simulink model "wlan_agc"  (Simulink 7.8)
settings: Solver=VariableStepDiscrete  SolverMode=SingleTasking  StartTime=0.0  StopTime=1e4  RelTol=1e-3
PostLoadFcn:
  | wlan_agc_init
InitFcn:
  | wlan_agc_init
StartFcn:
  | wlan_agc_init
undefined symbols (not defined in the file): gcbh, PHY_CONFIG_PKT_DET_CORR_THRESH, PHY_CONFIG_PKT_DET_ENERGY_THRESH, PHY_CONFIG_PKT_DET_MIN_DURR, xlBlockLoadCallback, xlGetNormalizedPeriod
libraries: xbsIndex_r4 x991, xbsEDKLib_r4 x1, simulink x1
(part 5 of 7)

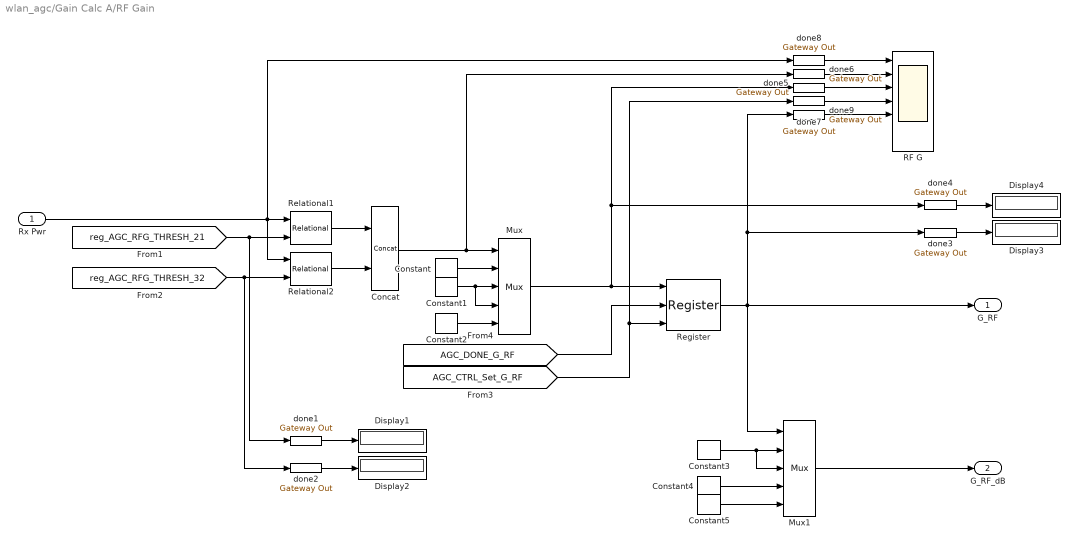
== system wlan_agc/Gain Calc A/RF Gain ==
  Rx Pwr : Inport
  Concat : xbsIndex_r4/Concat  num_inputs=2  dbl_ovrd=off  block_type=concat
  Constant : xbsIndex_r4/Constant  const=3  gui_display_data_type=Fixed-point  arith_type=Unsigned  n_bits=2  bin_pt=0  preci_type=Single  exp_width=8  frac_width=24  explicit_period=off  period=1  equ=P=C  opselect=C  inp2=PCIN>>17  opr=+  inp1=P  carry=CIN  dbl_ovrd=off  block_type=constant
  Constant1 : xbsIndex_r4/Constant  const=2  gui_display_data_type=Fixed-point  arith_type=Unsigned  n_bits=2  bin_pt=0  preci_type=Single  exp_width=8  frac_width=24  explicit_period=off  period=1  equ=P=C  opselect=C  inp2=PCIN>>17  opr=+  inp1=P  carry=CIN  dbl_ovrd=off  block_type=constant
  Constant2 : xbsIndex_r4/Constant  const=1  gui_display_data_type=Fixed-point  arith_type=Unsigned  n_bits=2  bin_pt=0  preci_type=Single  exp_width=8  frac_width=24  explicit_period=off  period=1  equ=P=C  opselect=C  inp2=PCIN>>17  opr=+  inp1=P  carry=CIN  dbl_ovrd=off  block_type=constant
  Constant3 : xbsIndex_r4/Constant  const=0  gui_display_data_type=Fixed-point  arith_type=Unsigned  n_bits=6  bin_pt=0  preci_type=Single  exp_width=8  frac_width=24  explicit_period=off  period=1  equ=P=C  opselect=C  inp2=PCIN>>17  opr=+  inp1=P  carry=CIN  dbl_ovrd=off  block_type=constant
  Constant4 : xbsIndex_r4/Constant  const=15  gui_display_data_type=Fixed-point  arith_type=Unsigned  n_bits=6  bin_pt=0  preci_type=Single  exp_width=8  frac_width=24  explicit_period=off  period=1  equ=P=C  opselect=C  inp2=PCIN>>17  opr=+  inp1=P  carry=CIN  dbl_ovrd=off  block_type=constant
  Constant5 : xbsIndex_r4/Constant  const=34  gui_display_data_type=Fixed-point  arith_type=Unsigned  n_bits=6  bin_pt=0  preci_type=Single  exp_width=8  frac_width=24  explicit_period=off  period=1  equ=P=C  opselect=C  inp2=PCIN>>17  opr=+  inp1=P  carry=CIN  dbl_ovrd=off  block_type=constant
  Display{1..4} (4 alike) : Display
  Mux : xbsIndex_r4/Mux  inputs=4  en=off  latency=0  precision=Full  arith_type=Unsigned  n_bits=16  bin_pt=14  quantization=Truncate  overflow=Wrap  dbl_ovrd=off  block_type=mux
  Mux1 : xbsIndex_r4/Mux  inputs=4  en=off  latency=0  precision=Full  arith_type=Unsigned  n_bits=16  bin_pt=14  quantization=Truncate  overflow=Wrap  dbl_ovrd=off  block_type=mux
  RF G : Scope  NumInputPorts=7
      settings: TimeRange=10000  YMin=-1~-1~0~0~0~-40~-1  YMax=1~1~0.8~0.2~80~0~1  SaveName=ScopeData5
  Register : xbsIndex_r4/Register  init=3  rst=on  en=on  dbl_ovrd=off  block_type=register
  Relational1 : xbsIndex_r4/Relational  mode=a>=b  en=off  latency=0  dbl_ovrd=off  block_type=relational
  Relational2 : xbsIndex_r4/Relational  mode=a>=b  en=off  latency=0  dbl_ovrd=off  block_type=relational
  done{1..9} (9 alike) : xbsIndex_r4/Gateway Out  inherit_from_input=off  hdl_port=off  timing_constraint=None  locs_specified=off  LOCs={}  UseAsDAC=off  DACChannel='1'  block_type=gatewayout
      settings: infoedit="Gateway out block.  Converts Xilinx fixed point inputs into ouputs of type Simulink integer, double, or fixed point.<P><P>Hardware notes:  In hardware these blocks become top level output ports or are discarded, depending on how they are configured."  xl_area=[0 0 0 0 1 0 0]  block_version=VER_STRING_GOES_HERE
  G_RF : Outport
  G_RF_dB : Outport  Port=2
  wires:
  Rx Pwr/1 -> Relational1/1, Relational2/1, done8/1
  [reg_AGC_RFG_THRESH_21] -> Relational1/2, done1/1
  Relational1/1 -> Concat/1
  [reg_AGC_RFG_THRESH_32] -> Relational2/2, done2/1
  Relational2/1 -> Concat/2
  Concat/1 -> Mux/1, done6/1
  Constant/1 -> Mux/2
  Constant1/1 -> Mux/3, Mux/4
  Constant2/1 -> Mux/5
  Mux/1 -> Register/1, done4/1, done5/1
  [AGC_DONE_G_RF] -> Register/2
  Register/1 -> G_RF/1, Mux1/1, done3/1, done9/1
  [AGC_CTRL_Set_G_RF] -> Register/3, done7/1
  Constant3/1 -> Mux1/2, Mux1/3
  Constant4/1 -> Mux1/4
  Constant5/1 -> Mux1/5
  Mux1/1 -> G_RF_dB/1
  done1/1 -> Display1/1
  done2/1 -> Display2/1
  done3/1 -> Display3/1
  done4/1 -> Display4/1
  done8/1 -> RF G/1
  done6/1 -> RF G/2
  done5/1 -> RF G/3
  done7/1 -> RF G/4
  done9/1 -> RF G/5

== system wlan_agc/Gain Calc A/RSSI Avg ==
  note: Flush recursive sum whenever sum
      | length changes. Otherwise let it run
      | (overflow is impossible, and lower
      | latency here is helpful to AGC timing)
  RSSI : Inport
  ASR : xbsIndex_r4/Addressable Shift Register  infer_latency=on  depth=2  initVector=[0]  en=off  dbl_ovrd=off  use_behavioral_HDL=off  Optimization=Resource  use_rpm=off  block_type=addrsr
      settings: infoedit="Delay of configurable length.  Any element in the delay line can be addressed and driven onto the output port.<br><br>Hardware notes: This block is implemented using SRL16s. If Virtex-4 or Spartan-3 device is used, multiple SRLC16s are cascaded together."  block_version=VER_STRING_GOES_HERE
  Accumulator : xbsIndex_r4/Accumulator  operation=Add  n_bits=16  overflow=Flag as error  scale=1  rst=on  infoeditControl=reset for floating point data type must be asserted for a minimum of 2 cycles  hasbypass=off  en=off  latency=0  dbl_ovrd=off  msb_inp=100  msb=100  lsb=-100  use_behavioral_HDL=on  implementation=Fabric  block_type=accum
      settings: block_version=VER_STRING_GOES_HERE
  AddSub : xbsIndex_r4/AddSub  mode=Subtraction  use_carryin=off  use_carryout=off  en=off  latency=0  precision=Full  arith_type=Unsigned  n_bits=10  bin_pt=0  quantization=Truncate  overflow=Wrap  dbl_ovrd=off  use_behavioral_HDL=off  hw_selection=Fabric  pipelined=off  use_rpm=on  block_type=addsub
      settings: block_version=VER_STRING_GOES_HERE
  Constant : xbsIndex_r4/Constant  const=0  gui_display_data_type=Fixed-point  arith_type=Unsigned  n_bits=2  bin_pt=0  preci_type=Single  exp_width=8  frac_width=24  explicit_period=off  period=1  equ=P=C  opselect=C  inp2=PCIN>>17  opr=+  inp1=P  carry=CIN  dbl_ovrd=off  block_type=constant
  Constant1 : xbsIndex_r4/Constant  const=1  gui_display_data_type=Fixed-point  arith_type=Unsigned  n_bits=2  bin_pt=0  preci_type=Single  exp_width=8  frac_width=24  explicit_period=off  period=1  equ=P=C  opselect=C  inp2=PCIN>>17  opr=+  inp1=P  carry=CIN  dbl_ovrd=off  block_type=constant
  Constant2 : xbsIndex_r4/Constant  const=3  gui_display_data_type=Fixed-point  arith_type=Unsigned  n_bits=3  bin_pt=0  preci_type=Single  exp_width=8  frac_width=24  explicit_period=off  period=1  equ=P=C  opselect=C  inp2=PCIN>>17  opr=+  inp1=P  carry=CIN  dbl_ovrd=off  block_type=constant
  Constant3 : xbsIndex_r4/Constant  const=7  gui_display_data_type=Fixed-point  arith_type=Unsigned  n_bits=3  bin_pt=0  preci_type=Single  exp_width=8  frac_width=24  explicit_period=off  period=1  equ=P=C  opselect=C  inp2=PCIN>>17  opr=+  inp1=P  carry=CIN  dbl_ovrd=off  block_type=constant
  Convert1 : xbsIndex_r4/Convert  gui_display_data_type=Fixed-point  arith_type=Unsigned  n_bits=10  bin_pt=0  float_type=Single  exp_bits=8  fraction_bits=24  quantization=Truncate  overflow=Saturate  en=off  latency=0  dbl_ovrd=off  pipeline=off  block_type=convert
      settings: block_version=10.1.3
  Down Sample1 : xbsIndex_r4/Down Sample  sample_ratio=16  sample_phase="Last Value of Frame  (most efficient)"  en=off  latency=1  dbl_ovrd=off  block_type=dsamp
  Mux : xbsIndex_r4/Mux  inputs=4  en=off  latency=0  precision=Full  arith_type=Unsigned  n_bits=16  bin_pt=14  quantization=Truncate  overflow=Wrap  dbl_ovrd=off  block_type=mux
  Mux1 : xbsIndex_r4/Mux  inputs=4  en=off  latency=0  precision=Full  arith_type=Unsigned  n_bits=16  bin_pt=14  quantization=Truncate  overflow=Wrap  dbl_ovrd=off  block_type=mux
  RSSI Avg : Scope  NumInputPorts=7
      settings: TimeRange=10000  YMin=0~0~0~0~0~-1~-1  YMax=1000~2~1~4000~1000~1~1  SaveName=ScopeData2
  Register : xbsIndex_r4/Register  init=0  rst=on  en=off  dbl_ovrd=off  block_type=register
      settings: block_version=VER_STRING_GOES_HERE
  Reset : Subsystem
  Shift : xbsIndex_r4/Shift  shift_dir=Right  shift_bits=1  en=off  latency=0  precision=Full  arith_type="Signed  (2's comp)"  n_bits=16  bin_pt=14  quantization=Truncate  overflow=Wrap  dbl_ovrd=off  block_type=shift
  Shift1 : xbsIndex_r4/Shift  shift_dir=Right  shift_bits=2  en=off  latency=0  precision=Full  arith_type="Signed  (2's comp)"  n_bits=16  bin_pt=14  quantization=Truncate  overflow=Wrap  dbl_ovrd=off  block_type=shift
  Shift2 : xbsIndex_r4/Shift  shift_dir=Right  shift_bits=3  en=off  latency=0  precision=Full  arith_type="Signed  (2's comp)"  n_bits=16  bin_pt=14  quantization=Truncate  overflow=Wrap  dbl_ovrd=off  block_type=shift
  done{2..6} (5 alike) : xbsIndex_r4/Gateway Out  inherit_from_input=off  hdl_port=off  timing_constraint=None  locs_specified=off  LOCs={}  UseAsDAC=off  DACChannel='1'  block_type=gatewayout
      settings: infoedit="Gateway out block.  Converts Xilinx fixed point inputs into ouputs of type Simulink integer, double, or fixed point.<P><P>Hardware notes:  In hardware these blocks become top level output ports or are discarded, depending on how they are configured."  xl_area=[0 0 0 0 1 0 0]  block_version=VER_STRING_GOES_HERE
  avg : Outport
  wires:
  ASR/1 -> AddSub/2
  AddSub/1 -> Accumulator/1
  Register/1 -> ASR/1, AddSub/1
  RSSI/1 -> Register/1, done4/1
  Accumulator/1 -> Mux1/2, Shift/1, Shift1/1, Shift2/1, done3/1
  Constant/1 -> Mux/2
  Constant1/1 -> Mux/3
  Constant2/1 -> Mux/4
  [reg_RSSI_AVG_LEN_SEL] -> Down Sample1/1, Mux1/1
  Constant3/1 -> Mux/5
  Mux/1 -> ASR/2
  Shift/1 -> Mux1/3
  Shift1/1 -> Mux1/4
  Shift2/1 -> Mux1/5
  Mux1/1 -> Convert1/1
  Convert1/1 -> avg/1, done6/1
  Down Sample1/1 -> Mux/1, Reset/1(Start), done2/1
  Reset/1(Rst) -> Accumulator/2, Register/2, done5/1
  done4/1 -> RSSI Avg/1
  done2/1 -> RSSI Avg/2
  done6/1 -> RSSI Avg/5
  done5/1 -> RSSI Avg/3
  done3/1 -> RSSI Avg/4
  ? -> RSSI Avg/6
  ? -> RSSI Avg/7

== system wlan_agc/Gain Calc B/BB gain ==
  G_RF_dB : Inport
  P_IN_RSSI : Inport  Port=2
  IQ_dBv : Inport  Port=3
  AddSub : xbsIndex_r4/AddSub  mode=Subtraction  use_carryin=off  use_carryout=off  en=off  latency=1  precision=User Defined  arith_type="Signed  (2's comp)"  n_bits=8  bin_pt=0  quantization=Truncate  overflow=Wrap  dbl_ovrd=off  use_behavioral_HDL=off  hw_selection=Fabric  pipelined=off  block_type=addsub
  AddSub1 : xbsIndex_r4/AddSub  mode=Subtraction  use_carryin=off  use_carryout=off  en=off  latency=1  precision=User Defined  arith_type="Signed  (2's comp)"  n_bits=8  bin_pt=0  quantization=Truncate  overflow=Wrap  dbl_ovrd=off  use_behavioral_HDL=off  hw_selection=Fabric  pipelined=off  block_type=addsub
  AddSub2 : xbsIndex_r4/AddSub  mode=Subtraction  use_carryin=off  use_carryout=off  en=off  latency=0  precision=User Defined  arith_type="Signed  (2's comp)"  n_bits=8  bin_pt=0  quantization=Truncate  overflow=Wrap  dbl_ovrd=off  use_behavioral_HDL=off  hw_selection=Fabric  pipelined=off  block_type=addsub
  AddSub3 : xbsIndex_r4/AddSub  mode=Addition  use_carryin=off  use_carryout=off  en=off  latency=1  precision=User Defined  arith_type="Signed  (2's comp)"  n_bits=8  bin_pt=0  quantization=Truncate  overflow=Wrap  dbl_ovrd=off  use_behavioral_HDL=off  hw_selection=Fabric  pipelined=off  block_type=addsub
  AddSub4 : xbsIndex_r4/AddSub  mode=Subtraction  use_carryin=off  use_carryout=off  en=off  latency=0  precision=User Defined  arith_type="Signed  (2's comp)"  n_bits=8  bin_pt=0  quantization=Truncate  overflow=Wrap  dbl_ovrd=off  use_behavioral_HDL=off  hw_selection=Fabric  pipelined=off  block_type=addsub
  Convert1 : xbsIndex_r4/Convert  gui_display_data_type=Fixed-point  arith_type=Unsigned  n_bits=5  bin_pt=0  float_type=Single  exp_bits=8  fraction_bits=24  quantization=Truncate  overflow=Saturate  en=off  latency=0  dbl_ovrd=off  pipeline=off  block_type=convert
  Convert2 : xbsIndex_r4/Convert  gui_display_data_type=Fixed-point  arith_type=Unsigned  n_bits=5  bin_pt=0  float_type=Single  exp_bits=8  fraction_bits=24  quantization=Truncate  overflow=Saturate  en=off  latency=0  dbl_ovrd=off  pipeline=off  block_type=convert
  Mux : xbsIndex_r4/Mux  inputs=3  en=off  latency=0  precision=Full  arith_type=Unsigned  n_bits=16  bin_pt=14  quantization=Truncate  overflow=Wrap  dbl_ovrd=off  block_type=mux
  Shift : xbsIndex_r4/Shift  shift_dir=Right  shift_bits=1  en=off  latency=0  precision=Full  arith_type="Signed  (2's comp)"  n_bits=16  bin_pt=14  quantization=Truncate  overflow=Wrap  dbl_ovrd=off  block_type=shift
  Shift1 : xbsIndex_r4/Shift  shift_dir=Right  shift_bits=1  en=off  latency=0  precision=Full  arith_type="Signed  (2's comp)"  n_bits=16  bin_pt=14  quantization=Truncate  overflow=Wrap  dbl_ovrd=off  block_type=shift
  G_BB : Outport
  wires:
  [reg_AGC_V_DB_ADJ] -> AddSub4/2
  IQ_dBv/1 -> AddSub4/1
  [AGC_CTRL_G_BB_SEL] -> Mux/1
  AddSub4/1 -> AddSub2/2
  P_IN_RSSI/1 -> AddSub/2
  Mux/1 -> G_BB/1
  G_RF_dB/1 -> AddSub1/2
  Convert2/1 -> Mux/4
  Convert1/1 -> Mux/3
  Shift1/1 -> Convert2/1
  AddSub3/1 -> Shift1/1
  AddSub2/1 -> AddSub3/1
  Shift/1 -> Convert1/1
  AddSub1/1 -> AddSub3/2, Shift/1
  AddSub/1 -> AddSub1/1
  [reg_AGC_TARGET_PWR] -> AddSub2/1, AddSub/1
  [reg_AGC_INIT_G_BB] -> Mux/2

== system wlan_agc/Gain Calc B/Capture & Convert ==
  note: Shift slope-adjusted value by gain-dependent
      | offset (top-center plot on pg 16 of MAX2829 ds)
  G_RF : Inport
  RSSI : Inport  Port=2
  AddSub : xbsIndex_r4/AddSub  mode=Subtraction  use_carryin=off  use_carryout=off  en=off  latency=1  precision=User Defined  arith_type="Signed  (2's comp)"  n_bits=8  bin_pt=0  quantization=Truncate  overflow=Flag as error  dbl_ovrd=off  use_behavioral_HDL=off  hw_selection=Fabric  pipelined=off  block_type=addsub
  Constant : xbsIndex_r4/Constant  const=1/15  gui_display_data_type=Fixed-point  arith_type=Unsigned  n_bits=12  bin_pt=12  preci_type=Single  exp_width=8  frac_width=24  explicit_period=off  period=1  equ=P=C  opselect=C  inp2=PCIN>>17  opr=+  inp1=P  carry=CIN  dbl_ovrd=off  block_type=constant
  Constant1 : xbsIndex_r4/Constant  const=100  gui_display_data_type=Fixed-point  arith_type=Unsigned  n_bits=7  bin_pt=0  preci_type=Single  exp_width=8  frac_width=24  explicit_period=off  period=1  equ=P=C  opselect=C  inp2=PCIN>>17  opr=+  inp1=P  carry=CIN  dbl_ovrd=off  block_type=constant
  Constant2 : xbsIndex_r4/Constant  const=85  gui_display_data_type=Fixed-point  arith_type=Unsigned  n_bits=7  bin_pt=0  preci_type=Single  exp_width=8  frac_width=24  explicit_period=off  period=1  equ=P=C  opselect=C  inp2=PCIN>>17  opr=+  inp1=P  carry=CIN  dbl_ovrd=off  block_type=constant
  Constant3 : xbsIndex_r4/Constant  const=70  gui_display_data_type=Fixed-point  arith_type=Unsigned  n_bits=7  bin_pt=0  preci_type=Single  exp_width=8  frac_width=24  explicit_period=off  period=1  equ=P=C  opselect=C  inp2=PCIN>>17  opr=+  inp1=P  carry=CIN  dbl_ovrd=off  block_type=constant
  Display : Display
  Display1 : Display
  Display2 : Display
  Mult : xbsIndex_r4/Mult  precision=User Defined  arith_type=Unsigned  n_bits=11  bin_pt=4  quantization=Truncate  overflow=Wrap  en=off  latency=1  dbl_ovrd=off  use_behavioral_HDL=off  opt=Speed  use_embedded=on  optimum_pipeline=off  pipeline=on  use_rpm=on  placement_style=Triangular  block_type=mult
  Mux1 : xbsIndex_r4/Mux  inputs=4  en=off  latency=0  precision=Full  arith_type=Unsigned  n_bits=16  bin_pt=14  quantization=Truncate  overflow=Wrap  dbl_ovrd=off  block_type=mux
  RSSI Calc : Scope  NumInputPorts=7
      settings: TimeRange=10000  YMin=-1~-1~0~0~0~-40~-1  YMax=1~1~0.8~0.2~80~0~1  SaveName=ScopeData7
  Register : xbsIndex_r4/Register  init=3  rst=on  en=on  dbl_ovrd=off  block_type=register
  done{1..8} (8 alike) : xbsIndex_r4/Gateway Out  inherit_from_input=off  hdl_port=off  timing_constraint=None  locs_specified=off  LOCs={}  UseAsDAC=off  DACChannel='1'  block_type=gatewayout
      settings: infoedit="Gateway out block.  Converts Xilinx fixed point inputs into ouputs of type Simulink integer, double, or fixed point.<P><P>Hardware notes:  In hardware these blocks become top level output ports or are discarded, depending on how they are configured."  xl_area=[0 0 0 0 1 0 0]  block_version=VER_STRING_GOES_HERE
  Rx Pwr (dBm) : Outport
  wires:
  done8/1 -> RSSI Calc/5
  done6/1 -> RSSI Calc/4
  done3/1 -> RSSI Calc/3
  done5/1 -> RSSI Calc/2
  done7/1 -> RSSI Calc/1
  done2/1 -> Display2/1
  done1/1 -> Display1/1
  done4/1 -> Display/1
  G_RF/1 -> Mux1/1
  [reg_AGC_RSSI_CALIB_G3] -> Mux1/5
  [reg_AGC_RSSI_CALIB_G2] -> Mux1/4
  [reg_AGC_RSSI_CALIB_G1] -> Mux1/3, Mux1/2
  AddSub/1 -> done8/1, done2/1, Rx Pwr (dBm)/1
  Mux1/1 -> done6/1, AddSub/2
  Mult/1 -> done4/1, AddSub/1
  Constant/1 -> Mult/2
  Register/1 -> done3/1, done1/1, Mult/1
  RSSI/1 -> done7/1, Register/1
  [AGC_RESET] -> Register/2
  [AGC_CTRL_Capture_RSSI] -> done5/1, Register/3

== system wlan_agc/Gain Calc B/IQ Mag ==
  I : Inport
  Q : Inport  Port=2
  Valid : Inport  Port=3
  AddSub : xbsIndex_r4/AddSub  mode=Addition  use_carryin=off  use_carryout=off  en=off  latency=0  precision=User Defined  arith_type=Unsigned  n_bits=20  bin_pt=19  quantization=Truncate  overflow=Flag as error  dbl_ovrd=off  use_behavioral_HDL=off  hw_selection=Fabric  pipelined=off  block_type=addsub
  Delay : xbsIndex_r4/Delay  rst=off  infoeditControl=Selection of Reset will increase slice count due to use of real FFs and instead of SRLs  en=off  latency=1  dbl_ovrd=off  reg_retiming=off  block_type=delay
  Mult : xbsIndex_r4/Mult  precision=User Defined  arith_type=Unsigned  n_bits=20  bin_pt=20  quantization=Truncate  overflow=Saturate  en=off  latency=1  dbl_ovrd=off  use_behavioral_HDL=off  opt=Speed  use_embedded=on  optimum_pipeline=off  pipeline=on  use_rpm=on  placement_style=Triangular  block_type=mult
  Mult1 : xbsIndex_r4/Mult  precision=User Defined  arith_type=Unsigned  n_bits=20  bin_pt=20  quantization=Truncate  overflow=Saturate  en=off  latency=1  dbl_ovrd=off  use_behavioral_HDL=off  opt=Speed  use_embedded=on  optimum_pipeline=off  pipeline=on  use_rpm=on  placement_style=Triangular  block_type=mult
  ROM : xbsIndex_r4/ROM  depth=2^11  initVector=5*log10(linspace(2^-11, 2, 2048))  distributed_mem=Block RAM  rst=off  init_reg=0  en=off  latency=1  gui_display_data_type=Fixed-point  arith_type="Signed  (2's comp)"  n_bits=14  bin_pt=8  preci_type=Single  exp_width=8  frac_width=24  dbl_ovrd=off  optimize=Area  use_rpm=on  block_type=sprom
  Register : xbsIndex_r4/Register  init=0  rst=on  en=on  dbl_ovrd=off  block_type=register
  Reinterpret : xbsIndex_r4/Reinterpret  force_arith_type=off  arith_type=Unsigned  force_bin_pt=on  bin_pt=0  block_type=reinterpret
  Running Sum : Subsystem
  V_DB : Scope  NumInputPorts=7
      settings: TimeRange=10000  YMin=-0.75~-0.75~0~0~0~-17.5~-1  YMax=0.75~0.75~0.35~0.125~125~0~1  SaveName=ScopeData4
  done{1..7} (7 alike) : xbsIndex_r4/Gateway Out  inherit_from_input=off  hdl_port=off  timing_constraint=None  locs_specified=off  LOCs={}  UseAsDAC=off  DACChannel='1'  block_type=gatewayout
      settings: infoedit="Gateway out block.  Converts Xilinx fixed point inputs into ouputs of type Simulink integer, double, or fixed point.<P><P>Hardware notes:  In hardware these blocks become top level output ports or are discarded, depending on how they are configured."  xl_area=[0 0 0 0 1 0 0]  block_version=VER_STRING_GOES_HERE
  IQ_dBv : Outport
  wires:
  done7/1 -> V_DB/7
  done6/1 -> V_DB/6
  done5/1 -> V_DB/5
  done3/1 -> V_DB/4
  done1/1 -> V_DB/3
  done2/1 -> V_DB/2
  done4/1 -> V_DB/1
  Reinterpret/1 -> done5/1, ROM/1
  Register/1 -> IQ_dBv/1
  [AGC_DONE_G_BB] -> Register/2
  [AGC_CTRL_Capture_V_DB] -> done7/1, Register/3
  ROM/1 -> done6/1, Register/1
  AddSub/1 -> done1/1, Running Sum/2(D)
  Mult1/1 -> AddSub/2
  Mult/1 -> AddSub/1
  Q/1 -> done2/1, Mult1/1, Mult1/2
  Running Sum/1(Sum) -> done3/1, Reinterpret/1
  Valid/1 -> Delay/1
  I/1 -> done4/1, Mult/2, Mult/1
  Delay/1 -> Running Sum/1(En)

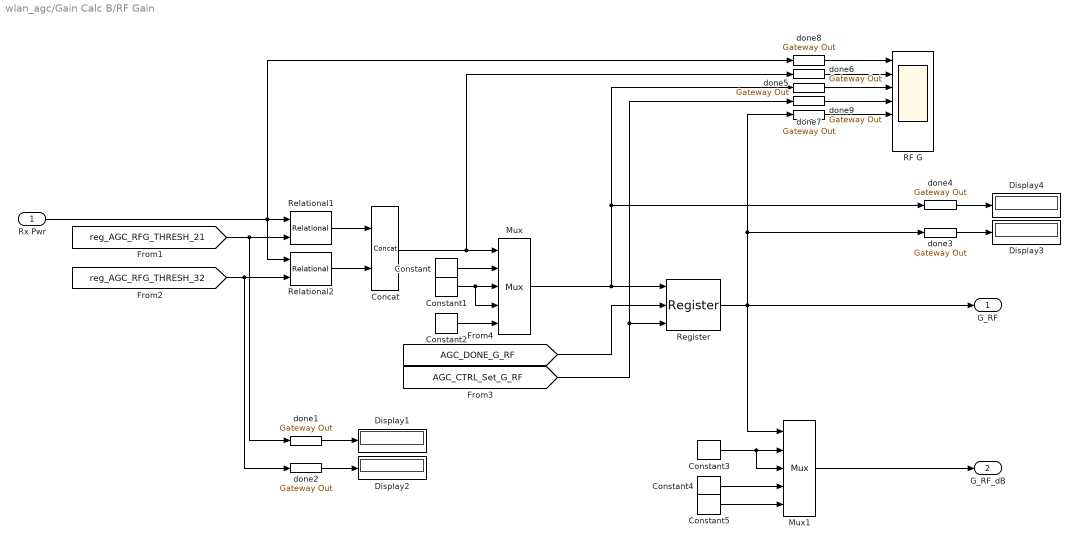
== system wlan_agc/Gain Calc B/RF Gain ==
  Rx Pwr : Inport
  Concat : xbsIndex_r4/Concat  num_inputs=2  dbl_ovrd=off  block_type=concat
  Constant : xbsIndex_r4/Constant  const=3  gui_display_data_type=Fixed-point  arith_type=Unsigned  n_bits=2  bin_pt=0  preci_type=Single  exp_width=8  frac_width=24  explicit_period=off  period=1  equ=P=C  opselect=C  inp2=PCIN>>17  opr=+  inp1=P  carry=CIN  dbl_ovrd=off  block_type=constant
  Constant1 : xbsIndex_r4/Constant  const=2  gui_display_data_type=Fixed-point  arith_type=Unsigned  n_bits=2  bin_pt=0  preci_type=Single  exp_width=8  frac_width=24  explicit_period=off  period=1  equ=P=C  opselect=C  inp2=PCIN>>17  opr=+  inp1=P  carry=CIN  dbl_ovrd=off  block_type=constant
  Constant2 : xbsIndex_r4/Constant  const=1  gui_display_data_type=Fixed-point  arith_type=Unsigned  n_bits=2  bin_pt=0  preci_type=Single  exp_width=8  frac_width=24  explicit_period=off  period=1  equ=P=C  opselect=C  inp2=PCIN>>17  opr=+  inp1=P  carry=CIN  dbl_ovrd=off  block_type=constant
  Constant3 : xbsIndex_r4/Constant  const=0  gui_display_data_type=Fixed-point  arith_type=Unsigned  n_bits=6  bin_pt=0  preci_type=Single  exp_width=8  frac_width=24  explicit_period=off  period=1  equ=P=C  opselect=C  inp2=PCIN>>17  opr=+  inp1=P  carry=CIN  dbl_ovrd=off  block_type=constant
  Constant4 : xbsIndex_r4/Constant  const=15  gui_display_data_type=Fixed-point  arith_type=Unsigned  n_bits=6  bin_pt=0  preci_type=Single  exp_width=8  frac_width=24  explicit_period=off  period=1  equ=P=C  opselect=C  inp2=PCIN>>17  opr=+  inp1=P  carry=CIN  dbl_ovrd=off  block_type=constant
  Constant5 : xbsIndex_r4/Constant  const=34  gui_display_data_type=Fixed-point  arith_type=Unsigned  n_bits=6  bin_pt=0  preci_type=Single  exp_width=8  frac_width=24  explicit_period=off  period=1  equ=P=C  opselect=C  inp2=PCIN>>17  opr=+  inp1=P  carry=CIN  dbl_ovrd=off  block_type=constant
  Display{1..4} (4 alike) : Display
  Mux : xbsIndex_r4/Mux  inputs=4  en=off  latency=0  precision=Full  arith_type=Unsigned  n_bits=16  bin_pt=14  quantization=Truncate  overflow=Wrap  dbl_ovrd=off  block_type=mux
  Mux1 : xbsIndex_r4/Mux  inputs=4  en=off  latency=0  precision=Full  arith_type=Unsigned  n_bits=16  bin_pt=14  quantization=Truncate  overflow=Wrap  dbl_ovrd=off  block_type=mux
  RF G : Scope  NumInputPorts=7
      settings: TimeRange=10000  YMin=-1~-1~0~0~0~-40~-1  YMax=1~1~0.8~0.2~80~0~1  SaveName=ScopeData5
  Register : xbsIndex_r4/Register  init=3  rst=on  en=on  dbl_ovrd=off  block_type=register
  Relational1 : xbsIndex_r4/Relational  mode=a>=b  en=off  latency=0  dbl_ovrd=off  block_type=relational
  Relational2 : xbsIndex_r4/Relational  mode=a>=b  en=off  latency=0  dbl_ovrd=off  block_type=relational
  done{1..9} (9 alike) : xbsIndex_r4/Gateway Out  inherit_from_input=off  hdl_port=off  timing_constraint=None  locs_specified=off  LOCs={}  UseAsDAC=off  DACChannel='1'  block_type=gatewayout
      settings: infoedit="Gateway out block.  Converts Xilinx fixed point inputs into ouputs of type Simulink integer, double, or fixed point.<P><P>Hardware notes:  In hardware these blocks become top level output ports or are discarded, depending on how they are configured."  xl_area=[0 0 0 0 1 0 0]  block_version=VER_STRING_GOES_HERE
  G_RF : Outport
  G_RF_dB : Outport  Port=2
  wires:
  done9/1 -> RF G/5
  done7/1 -> RF G/4
  done5/1 -> RF G/3
  done6/1 -> RF G/2
  done8/1 -> RF G/1
  done4/1 -> Display4/1
  done3/1 -> Display3/1
  done2/1 -> Display2/1
  done1/1 -> Display1/1
  Mux1/1 -> G_RF_dB/1
  Constant5/1 -> Mux1/5
  Constant4/1 -> Mux1/4
  Constant3/1 -> Mux1/3, Mux1/2
  [AGC_CTRL_Set_G_RF] -> done7/1, Register/3
  Register/1 -> done9/1, done3/1, Mux1/1, G_RF/1
  [AGC_DONE_G_RF] -> Register/2
  Mux/1 -> done5/1, done4/1, Register/1
  Constant2/1 -> Mux/5
  Constant1/1 -> Mux/4, Mux/3
  Constant/1 -> Mux/2
  Concat/1 -> done6/1, Mux/1
  Relational2/1 -> Concat/2
  [reg_AGC_RFG_THRESH_32] -> done2/1, Relational2/2
  Relational1/1 -> Concat/1
  [reg_AGC_RFG_THRESH_21] -> done1/1, Relational1/2
  Rx Pwr/1 -> done8/1, Relational2/1, Relational1/1

== system wlan_agc/Gain Calc B/RSSI Avg ==
  note: Flush recursive sum whenever sum
      | length changes. Otherwise let it run
      | (overflow is impossible, and lower
      | latency here is helpful to AGC timing)
  RSSI : Inport
  ASR : xbsIndex_r4/Addressable Shift Register  infer_latency=on  depth=2  initVector=[0]  en=off  dbl_ovrd=off  use_behavioral_HDL=off  Optimization=Resource  use_rpm=off  block_type=addrsr
      settings: infoedit="Delay of configurable length.  Any element in the delay line can be addressed and driven onto the output port.<br><br>Hardware notes: This block is implemented using SRL16s. If Virtex-4 or Spartan-3 device is used, multiple SRLC16s are cascaded together."  block_version=VER_STRING_GOES_HERE
  Accumulator : xbsIndex_r4/Accumulator  operation=Add  n_bits=16  overflow=Flag as error  scale=1  rst=on  infoeditControl=reset for floating point data type must be asserted for a minimum of 2 cycles  hasbypass=off  en=off  latency=0  dbl_ovrd=off  msb_inp=100  msb=100  lsb=-100  use_behavioral_HDL=on  implementation=Fabric  block_type=accum
      settings: block_version=VER_STRING_GOES_HERE
  AddSub : xbsIndex_r4/AddSub  mode=Subtraction  use_carryin=off  use_carryout=off  en=off  latency=0  precision=Full  arith_type=Unsigned  n_bits=10  bin_pt=0  quantization=Truncate  overflow=Wrap  dbl_ovrd=off  use_behavioral_HDL=off  hw_selection=Fabric  pipelined=off  use_rpm=on  block_type=addsub
      settings: block_version=VER_STRING_GOES_HERE
  Constant : xbsIndex_r4/Constant  const=0  gui_display_data_type=Fixed-point  arith_type=Unsigned  n_bits=2  bin_pt=0  preci_type=Single  exp_width=8  frac_width=24  explicit_period=off  period=1  equ=P=C  opselect=C  inp2=PCIN>>17  opr=+  inp1=P  carry=CIN  dbl_ovrd=off  block_type=constant
  Constant1 : xbsIndex_r4/Constant  const=1  gui_display_data_type=Fixed-point  arith_type=Unsigned  n_bits=2  bin_pt=0  preci_type=Single  exp_width=8  frac_width=24  explicit_period=off  period=1  equ=P=C  opselect=C  inp2=PCIN>>17  opr=+  inp1=P  carry=CIN  dbl_ovrd=off  block_type=constant
  Constant2 : xbsIndex_r4/Constant  const=3  gui_display_data_type=Fixed-point  arith_type=Unsigned  n_bits=3  bin_pt=0  preci_type=Single  exp_width=8  frac_width=24  explicit_period=off  period=1  equ=P=C  opselect=C  inp2=PCIN>>17  opr=+  inp1=P  carry=CIN  dbl_ovrd=off  block_type=constant
  Constant3 : xbsIndex_r4/Constant  const=7  gui_display_data_type=Fixed-point  arith_type=Unsigned  n_bits=3  bin_pt=0  preci_type=Single  exp_width=8  frac_width=24  explicit_period=off  period=1  equ=P=C  opselect=C  inp2=PCIN>>17  opr=+  inp1=P  carry=CIN  dbl_ovrd=off  block_type=constant
  Convert1 : xbsIndex_r4/Convert  gui_display_data_type=Fixed-point  arith_type=Unsigned  n_bits=10  bin_pt=0  float_type=Single  exp_bits=8  fraction_bits=24  quantization=Truncate  overflow=Saturate  en=off  latency=0  dbl_ovrd=off  pipeline=off  block_type=convert
      settings: block_version=10.1.3
  Down Sample1 : xbsIndex_r4/Down Sample  sample_ratio=16  sample_phase="Last Value of Frame  (most efficient)"  en=off  latency=1  dbl_ovrd=off  block_type=dsamp
  Mux : xbsIndex_r4/Mux  inputs=4  en=off  latency=0  precision=Full  arith_type=Unsigned  n_bits=16  bin_pt=14  quantization=Truncate  overflow=Wrap  dbl_ovrd=off  block_type=mux
  Mux1 : xbsIndex_r4/Mux  inputs=4  en=off  latency=0  precision=Full  arith_type=Unsigned  n_bits=16  bin_pt=14  quantization=Truncate  overflow=Wrap  dbl_ovrd=off  block_type=mux
  RSSI Avg : Scope  NumInputPorts=7
      settings: TimeRange=10000  YMin=0~0~0~0~0~-1~-1  YMax=1000~2~1~4000~1000~1~1  SaveName=ScopeData2
  Register : xbsIndex_r4/Register  init=0  rst=on  en=off  dbl_ovrd=off  block_type=register
      settings: block_version=VER_STRING_GOES_HERE
  Reset : Subsystem
  Shift : xbsIndex_r4/Shift  shift_dir=Right  shift_bits=1  en=off  latency=0  precision=Full  arith_type="Signed  (2's comp)"  n_bits=16  bin_pt=14  quantization=Truncate  overflow=Wrap  dbl_ovrd=off  block_type=shift
  Shift1 : xbsIndex_r4/Shift  shift_dir=Right  shift_bits=2  en=off  latency=0  precision=Full  arith_type="Signed  (2's comp)"  n_bits=16  bin_pt=14  quantization=Truncate  overflow=Wrap  dbl_ovrd=off  block_type=shift
  Shift2 : xbsIndex_r4/Shift  shift_dir=Right  shift_bits=3  en=off  latency=0  precision=Full  arith_type="Signed  (2's comp)"  n_bits=16  bin_pt=14  quantization=Truncate  overflow=Wrap  dbl_ovrd=off  block_type=shift
  done{2..6} (5 alike) : xbsIndex_r4/Gateway Out  inherit_from_input=off  hdl_port=off  timing_constraint=None  locs_specified=off  LOCs={}  UseAsDAC=off  DACChannel='1'  block_type=gatewayout
      settings: infoedit="Gateway out block.  Converts Xilinx fixed point inputs into ouputs of type Simulink integer, double, or fixed point.<P><P>Hardware notes:  In hardware these blocks become top level output ports or are discarded, depending on how they are configured."  xl_area=[0 0 0 0 1 0 0]  block_version=VER_STRING_GOES_HERE
  avg : Outport
  wires:
  ? -> RSSI Avg/7
  ? -> RSSI Avg/6
  done3/1 -> RSSI Avg/4
  done5/1 -> RSSI Avg/3
  done6/1 -> RSSI Avg/5
  done2/1 -> RSSI Avg/2
  done4/1 -> RSSI Avg/1
  Reset/1(Rst) -> done5/1, Register/2, Accumulator/2
  Down Sample1/1 -> done2/1, Reset/1(Start), Mux/1
  Convert1/1 -> done6/1, avg/1
  Mux1/1 -> Convert1/1
  Shift2/1 -> Mux1/5
  Shift1/1 -> Mux1/4
  Shift/1 -> Mux1/3
  Mux/1 -> ASR/2
  Constant3/1 -> Mux/5
  [reg_RSSI_AVG_LEN_SEL] -> Mux1/1, Down Sample1/1
  Constant2/1 -> Mux/4
  Constant1/1 -> Mux/3
  Constant/1 -> Mux/2
  Accumulator/1 -> done3/1, Shift2/1, Shift1/1, Shift/1, Mux1/2
  RSSI/1 -> done4/1, Register/1
  Register/1 -> AddSub/1, ASR/1
  AddSub/1 -> Accumulator/1
  ASR/1 -> AddSub/2

== system wlan_agc/Gain Calc C/BB gain ==
  G_RF_dB : Inport
  P_IN_RSSI : Inport  Port=2
  IQ_dBv : Inport  Port=3
  AddSub : xbsIndex_r4/AddSub  mode=Subtraction  use_carryin=off  use_carryout=off  en=off  latency=1  precision=User Defined  arith_type="Signed  (2's comp)"  n_bits=8  bin_pt=0  quantization=Truncate  overflow=Wrap  dbl_ovrd=off  use_behavioral_HDL=off  hw_selection=Fabric  pipelined=off  block_type=addsub
  AddSub1 : xbsIndex_r4/AddSub  mode=Subtraction  use_carryin=off  use_carryout=off  en=off  latency=1  precision=User Defined  arith_type="Signed  (2's comp)"  n_bits=8  bin_pt=0  quantization=Truncate  overflow=Wrap  dbl_ovrd=off  use_behavioral_HDL=off  hw_selection=Fabric  pipelined=off  block_type=addsub
  AddSub2 : xbsIndex_r4/AddSub  mode=Subtraction  use_carryin=off  use_carryout=off  en=off  latency=0  precision=User Defined  arith_type="Signed  (2's comp)"  n_bits=8  bin_pt=0  quantization=Truncate  overflow=Wrap  dbl_ovrd=off  use_behavioral_HDL=off  hw_selection=Fabric  pipelined=off  block_type=addsub
  AddSub3 : xbsIndex_r4/AddSub  mode=Addition  use_carryin=off  use_carryout=off  en=off  latency=1  precision=User Defined  arith_type="Signed  (2's comp)"  n_bits=8  bin_pt=0  quantization=Truncate  overflow=Wrap  dbl_ovrd=off  use_behavioral_HDL=off  hw_selection=Fabric  pipelined=off  block_type=addsub
  AddSub4 : xbsIndex_r4/AddSub  mode=Subtraction  use_carryin=off  use_carryout=off  en=off  latency=0  precision=User Defined  arith_type="Signed  (2's comp)"  n_bits=8  bin_pt=0  quantization=Truncate  overflow=Wrap  dbl_ovrd=off  use_behavioral_HDL=off  hw_selection=Fabric  pipelined=off  block_type=addsub
  Convert1 : xbsIndex_r4/Convert  gui_display_data_type=Fixed-point  arith_type=Unsigned  n_bits=5  bin_pt=0  float_type=Single  exp_bits=8  fraction_bits=24  quantization=Truncate  overflow=Saturate  en=off  latency=0  dbl_ovrd=off  pipeline=off  block_type=convert
  Convert2 : xbsIndex_r4/Convert  gui_display_data_type=Fixed-point  arith_type=Unsigned  n_bits=5  bin_pt=0  float_type=Single  exp_bits=8  fraction_bits=24  quantization=Truncate  overflow=Saturate  en=off  latency=0  dbl_ovrd=off  pipeline=off  block_type=convert
  Mux : xbsIndex_r4/Mux  inputs=3  en=off  latency=0  precision=Full  arith_type=Unsigned  n_bits=16  bin_pt=14  quantization=Truncate  overflow=Wrap  dbl_ovrd=off  block_type=mux
  Shift : xbsIndex_r4/Shift  shift_dir=Right  shift_bits=1  en=off  latency=0  precision=Full  arith_type="Signed  (2's comp)"  n_bits=16  bin_pt=14  quantization=Truncate  overflow=Wrap  dbl_ovrd=off  block_type=shift
  Shift1 : xbsIndex_r4/Shift  shift_dir=Right  shift_bits=1  en=off  latency=0  precision=Full  arith_type="Signed  (2's comp)"  n_bits=16  bin_pt=14  quantization=Truncate  overflow=Wrap  dbl_ovrd=off  block_type=shift
  G_BB : Outport
  wires:
  [reg_AGC_INIT_G_BB] -> Mux/2
  [reg_AGC_TARGET_PWR] -> AddSub/1, AddSub2/1
  AddSub/1 -> AddSub1/1
  AddSub1/1 -> Shift/1, AddSub3/2
  Shift/1 -> Convert1/1
  AddSub2/1 -> AddSub3/1
  AddSub3/1 -> Shift1/1
  Shift1/1 -> Convert2/1
  Convert1/1 -> Mux/3
  Convert2/1 -> Mux/4
  G_RF_dB/1 -> AddSub1/2
  Mux/1 -> G_BB/1
  P_IN_RSSI/1 -> AddSub/2
  AddSub4/1 -> AddSub2/2
  [AGC_CTRL_G_BB_SEL] -> Mux/1
  IQ_dBv/1 -> AddSub4/1
  [reg_AGC_V_DB_ADJ] -> AddSub4/2

== system wlan_agc/Gain Calc C/Capture & Convert ==
  note: Shift slope-adjusted value by gain-dependent
      | offset (top-center plot on pg 16 of MAX2829 ds)
  G_RF : Inport
  RSSI : Inport  Port=2
  AddSub : xbsIndex_r4/AddSub  mode=Subtraction  use_carryin=off  use_carryout=off  en=off  latency=1  precision=User Defined  arith_type="Signed  (2's comp)"  n_bits=8  bin_pt=0  quantization=Truncate  overflow=Flag as error  dbl_ovrd=off  use_behavioral_HDL=off  hw_selection=Fabric  pipelined=off  block_type=addsub
  Constant : xbsIndex_r4/Constant  const=1/15  gui_display_data_type=Fixed-point  arith_type=Unsigned  n_bits=12  bin_pt=12  preci_type=Single  exp_width=8  frac_width=24  explicit_period=off  period=1  equ=P=C  opselect=C  inp2=PCIN>>17  opr=+  inp1=P  carry=CIN  dbl_ovrd=off  block_type=constant
  Constant1 : xbsIndex_r4/Constant  const=100  gui_display_data_type=Fixed-point  arith_type=Unsigned  n_bits=7  bin_pt=0  preci_type=Single  exp_width=8  frac_width=24  explicit_period=off  period=1  equ=P=C  opselect=C  inp2=PCIN>>17  opr=+  inp1=P  carry=CIN  dbl_ovrd=off  block_type=constant
  Constant2 : xbsIndex_r4/Constant  const=85  gui_display_data_type=Fixed-point  arith_type=Unsigned  n_bits=7  bin_pt=0  preci_type=Single  exp_width=8  frac_width=24  explicit_period=off  period=1  equ=P=C  opselect=C  inp2=PCIN>>17  opr=+  inp1=P  carry=CIN  dbl_ovrd=off  block_type=constant
  Constant3 : xbsIndex_r4/Constant  const=70  gui_display_data_type=Fixed-point  arith_type=Unsigned  n_bits=7  bin_pt=0  preci_type=Single  exp_width=8  frac_width=24  explicit_period=off  period=1  equ=P=C  opselect=C  inp2=PCIN>>17  opr=+  inp1=P  carry=CIN  dbl_ovrd=off  block_type=constant
  Display : Display
  Display1 : Display
  Display2 : Display
  Mult : xbsIndex_r4/Mult  precision=User Defined  arith_type=Unsigned  n_bits=11  bin_pt=4  quantization=Truncate  overflow=Wrap  en=off  latency=1  dbl_ovrd=off  use_behavioral_HDL=off  opt=Speed  use_embedded=on  optimum_pipeline=off  pipeline=on  use_rpm=on  placement_style=Triangular  block_type=mult
  Mux1 : xbsIndex_r4/Mux  inputs=4  en=off  latency=0  precision=Full  arith_type=Unsigned  n_bits=16  bin_pt=14  quantization=Truncate  overflow=Wrap  dbl_ovrd=off  block_type=mux
  RSSI Calc : Scope  NumInputPorts=7
      settings: TimeRange=10000  YMin=-1~-1~0~0~0~-40~-1  YMax=1~1~0.8~0.2~80~0~1  SaveName=ScopeData7
  Register : xbsIndex_r4/Register  init=3  rst=on  en=on  dbl_ovrd=off  block_type=register
  done{1..8} (8 alike) : xbsIndex_r4/Gateway Out  inherit_from_input=off  hdl_port=off  timing_constraint=None  locs_specified=off  LOCs={}  UseAsDAC=off  DACChannel='1'  block_type=gatewayout
      settings: infoedit="Gateway out block.  Converts Xilinx fixed point inputs into ouputs of type Simulink integer, double, or fixed point.<P><P>Hardware notes:  In hardware these blocks become top level output ports or are discarded, depending on how they are configured."  xl_area=[0 0 0 0 1 0 0]  block_version=VER_STRING_GOES_HERE
  Rx Pwr (dBm) : Outport
  wires:
  [AGC_CTRL_Capture_RSSI] -> Register/3, done5/1
  [AGC_RESET] -> Register/2
  RSSI/1 -> Register/1, done7/1
  Register/1 -> Mult/1, done1/1, done3/1
  Constant/1 -> Mult/2
  Mult/1 -> AddSub/1, done4/1
  Mux1/1 -> AddSub/2, done6/1
  AddSub/1 -> Rx Pwr (dBm)/1, done2/1, done8/1
  [reg_AGC_RSSI_CALIB_G1] -> Mux1/2, Mux1/3
  [reg_AGC_RSSI_CALIB_G2] -> Mux1/4
  [reg_AGC_RSSI_CALIB_G3] -> Mux1/5
  G_RF/1 -> Mux1/1
  done4/1 -> Display/1
  done1/1 -> Display1/1
  done2/1 -> Display2/1
  done7/1 -> RSSI Calc/1
  done5/1 -> RSSI Calc/2
  done3/1 -> RSSI Calc/3
  done6/1 -> RSSI Calc/4
  done8/1 -> RSSI Calc/5

== system wlan_agc/Gain Calc C/IQ Mag ==
  I : Inport
  Q : Inport  Port=2
  Valid : Inport  Port=3
  AddSub : xbsIndex_r4/AddSub  mode=Addition  use_carryin=off  use_carryout=off  en=off  latency=0  precision=User Defined  arith_type=Unsigned  n_bits=20  bin_pt=19  quantization=Truncate  overflow=Flag as error  dbl_ovrd=off  use_behavioral_HDL=off  hw_selection=Fabric  pipelined=off  block_type=addsub
  Delay : xbsIndex_r4/Delay  rst=off  infoeditControl=Selection of Reset will increase slice count due to use of real FFs and instead of SRLs  en=off  latency=1  dbl_ovrd=off  reg_retiming=off  block_type=delay
  Mult : xbsIndex_r4/Mult  precision=User Defined  arith_type=Unsigned  n_bits=20  bin_pt=20  quantization=Truncate  overflow=Saturate  en=off  latency=1  dbl_ovrd=off  use_behavioral_HDL=off  opt=Speed  use_embedded=on  optimum_pipeline=off  pipeline=on  use_rpm=on  placement_style=Triangular  block_type=mult
  Mult1 : xbsIndex_r4/Mult  precision=User Defined  arith_type=Unsigned  n_bits=20  bin_pt=20  quantization=Truncate  overflow=Saturate  en=off  latency=1  dbl_ovrd=off  use_behavioral_HDL=off  opt=Speed  use_embedded=on  optimum_pipeline=off  pipeline=on  use_rpm=on  placement_style=Triangular  block_type=mult
  ROM : xbsIndex_r4/ROM  depth=2^11  initVector=5*log10(linspace(2^-11, 2, 2048))  distributed_mem=Block RAM  rst=off  init_reg=0  en=off  latency=1  gui_display_data_type=Fixed-point  arith_type="Signed  (2's comp)"  n_bits=14  bin_pt=8  preci_type=Single  exp_width=8  frac_width=24  dbl_ovrd=off  optimize=Area  use_rpm=on  block_type=sprom
  Register : xbsIndex_r4/Register  init=0  rst=on  en=on  dbl_ovrd=off  block_type=register
  Reinterpret : xbsIndex_r4/Reinterpret  force_arith_type=off  arith_type=Unsigned  force_bin_pt=on  bin_pt=0  block_type=reinterpret
  Running Sum : Subsystem
  V_DB : Scope  NumInputPorts=7
      settings: TimeRange=10000  YMin=-0.75~-0.75~0~0~0~-17.5~-1  YMax=0.75~0.75~0.35~0.125~125~0~1  SaveName=ScopeData4
  done{1..7} (7 alike) : xbsIndex_r4/Gateway Out  inherit_from_input=off  hdl_port=off  timing_constraint=None  locs_specified=off  LOCs={}  UseAsDAC=off  DACChannel='1'  block_type=gatewayout
      settings: infoedit="Gateway out block.  Converts Xilinx fixed point inputs into ouputs of type Simulink integer, double, or fixed point.<P><P>Hardware notes:  In hardware these blocks become top level output ports or are discarded, depending on how they are configured."  xl_area=[0 0 0 0 1 0 0]  block_version=VER_STRING_GOES_HERE
  IQ_dBv : Outport
  wires:
  Delay/1 -> Running Sum/1(En)
  I/1 -> Mult/1, Mult/2, done4/1
  Valid/1 -> Delay/1
  Running Sum/1(Sum) -> Reinterpret/1, done3/1
  Q/1 -> Mult1/2, Mult1/1, done2/1
  Mult/1 -> AddSub/1
  Mult1/1 -> AddSub/2
  AddSub/1 -> Running Sum/2(D), done1/1
  ROM/1 -> Register/1, done6/1
  [AGC_CTRL_Capture_V_DB] -> Register/3, done7/1
  [AGC_DONE_G_BB] -> Register/2
  Register/1 -> IQ_dBv/1
  Reinterpret/1 -> ROM/1, done5/1
  done4/1 -> V_DB/1
  done2/1 -> V_DB/2
  done1/1 -> V_DB/3
  done3/1 -> V_DB/4
  done5/1 -> V_DB/5
  done6/1 -> V_DB/6
  done7/1 -> V_DB/7

== system wlan_agc/Gain Calc C/RF Gain ==
  Rx Pwr : Inport
  Concat : xbsIndex_r4/Concat  num_inputs=2  dbl_ovrd=off  block_type=concat
  Constant : xbsIndex_r4/Constant  const=3  gui_display_data_type=Fixed-point  arith_type=Unsigned  n_bits=2  bin_pt=0  preci_type=Single  exp_width=8  frac_width=24  explicit_period=off  period=1  equ=P=C  opselect=C  inp2=PCIN>>17  opr=+  inp1=P  carry=CIN  dbl_ovrd=off  block_type=constant
  Constant1 : xbsIndex_r4/Constant  const=2  gui_display_data_type=Fixed-point  arith_type=Unsigned  n_bits=2  bin_pt=0  preci_type=Single  exp_width=8  frac_width=24  explicit_period=off  period=1  equ=P=C  opselect=C  inp2=PCIN>>17  opr=+  inp1=P  carry=CIN  dbl_ovrd=off  block_type=constant
  Constant2 : xbsIndex_r4/Constant  const=1  gui_display_data_type=Fixed-point  arith_type=Unsigned  n_bits=2  bin_pt=0  preci_type=Single  exp_width=8  frac_width=24  explicit_period=off  period=1  equ=P=C  opselect=C  inp2=PCIN>>17  opr=+  inp1=P  carry=CIN  dbl_ovrd=off  block_type=constant
  Constant3 : xbsIndex_r4/Constant  const=0  gui_display_data_type=Fixed-point  arith_type=Unsigned  n_bits=6  bin_pt=0  preci_type=Single  exp_width=8  frac_width=24  explicit_period=off  period=1  equ=P=C  opselect=C  inp2=PCIN>>17  opr=+  inp1=P  carry=CIN  dbl_ovrd=off  block_type=constant
  Constant4 : xbsIndex_r4/Constant  const=15  gui_display_data_type=Fixed-point  arith_type=Unsigned  n_bits=6  bin_pt=0  preci_type=Single  exp_width=8  frac_width=24  explicit_period=off  period=1  equ=P=C  opselect=C  inp2=PCIN>>17  opr=+  inp1=P  carry=CIN  dbl_ovrd=off  block_type=constant
  Constant5 : xbsIndex_r4/Constant  const=34  gui_display_data_type=Fixed-point  arith_type=Unsigned  n_bits=6  bin_pt=0  preci_type=Single  exp_width=8  frac_width=24  explicit_period=off  period=1  equ=P=C  opselect=C  inp2=PCIN>>17  opr=+  inp1=P  carry=CIN  dbl_ovrd=off  block_type=constant
  Display{1..4} (4 alike) : Display
  Mux : xbsIndex_r4/Mux  inputs=4  en=off  latency=0  precision=Full  arith_type=Unsigned  n_bits=16  bin_pt=14  quantization=Truncate  overflow=Wrap  dbl_ovrd=off  block_type=mux
  Mux1 : xbsIndex_r4/Mux  inputs=4  en=off  latency=0  precision=Full  arith_type=Unsigned  n_bits=16  bin_pt=14  quantization=Truncate  overflow=Wrap  dbl_ovrd=off  block_type=mux
  RF G : Scope  NumInputPorts=7
      settings: TimeRange=10000  YMin=-1~-1~0~0~0~-40~-1  YMax=1~1~0.8~0.2~80~0~1  SaveName=ScopeData5
  Register : xbsIndex_r4/Register  init=3  rst=on  en=on  dbl_ovrd=off  block_type=register
  Relational1 : xbsIndex_r4/Relational  mode=a>=b  en=off  latency=0  dbl_ovrd=off  block_type=relational
  Relational2 : xbsIndex_r4/Relational  mode=a>=b  en=off  latency=0  dbl_ovrd=off  block_type=relational
  done{1..9} (9 alike) : xbsIndex_r4/Gateway Out  inherit_from_input=off  hdl_port=off  timing_constraint=None  locs_specified=off  LOCs={}  UseAsDAC=off  DACChannel='1'  block_type=gatewayout
      settings: infoedit="Gateway out block.  Converts Xilinx fixed point inputs into ouputs of type Simulink integer, double, or fixed point.<P><P>Hardware notes:  In hardware these blocks become top level output ports or are discarded, depending on how they are configured."  xl_area=[0 0 0 0 1 0 0]  block_version=VER_STRING_GOES_HERE
  G_RF : Outport
  G_RF_dB : Outport  Port=2
  wires:
  Rx Pwr/1 -> Relational1/1, Relational2/1, done8/1
  [reg_AGC_RFG_THRESH_21] -> Relational1/2, done1/1
  Relational1/1 -> Concat/1
  [reg_AGC_RFG_THRESH_32] -> Relational2/2, done2/1
  Relational2/1 -> Concat/2
  Concat/1 -> Mux/1, done6/1
  Constant/1 -> Mux/2
  Constant1/1 -> Mux/3, Mux/4
  Constant2/1 -> Mux/5
  Mux/1 -> Register/1, done4/1, done5/1
  [AGC_DONE_G_RF] -> Register/2
  Register/1 -> G_RF/1, Mux1/1, done3/1, done9/1
  [AGC_CTRL_Set_G_RF] -> Register/3, done7/1
  Constant3/1 -> Mux1/2, Mux1/3
  Constant4/1 -> Mux1/4
  Constant5/1 -> Mux1/5
  Mux1/1 -> G_RF_dB/1
  done1/1 -> Display1/1
  done2/1 -> Display2/1
  done3/1 -> Display3/1
  done4/1 -> Display4/1
  done8/1 -> RF G/1
  done6/1 -> RF G/2
  done5/1 -> RF G/3
  done7/1 -> RF G/4
  done9/1 -> RF G/5
